simulink model "TriggeredDiagram"  (R2015a)
settings: Solver=FixedStepDiscrete  SolverMode=SingleTasking  StartTime=0.0  StopTime=10.0  FixedStep=1  RelTol=1e-3
settings Model: CovMetricSettings=dwe  CovHtmlReporting=off  covSaveCumulativeToWorkspaceVar=off  CovSaveSingleToWorkspaceVar=off  CovExternalEMLEnable=on  Creator=hbourbou  LastModifiedBy=hbourbou
settings DataIOCC: LimitDataPoints=off  SaveFormat=Dataset
settings DebuggingCC: SFUnexpectedBacktrackingDiag=error  SFNoUnconditionalDefaultTransitionDiag=error
settings HardwareCC: ProdBitPerPointer=64  ProdLargestAtomicFloat=Float  ProdIntDivRoundTo=Zero  ProdEndianess=LittleEndian  ProdHWDeviceType=Specified
settings ModelReferenceCC: PropagateSignalLabelsOutOfModel=on
settings GRTTargetCC: TargetLangStandard=C99 (ISO)  GeneratePreprocessorConditionals=Use local settings

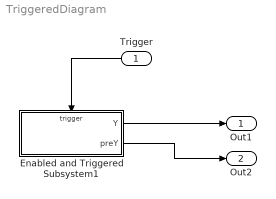
== system TriggeredDiagram ==
  Trigger : Inport  OutDataTypeStr=boolean
  Enabled and Triggered Subsystem1 : Subsystem  TreatAsAtomicUnit=on
  Out1 : Outport
  Out2 : Outport  Port=2
  wires:
  Enabled and Triggered Subsystem1/1(Y) -> Out1/1
  Enabled and Triggered Subsystem1/2(preY) -> Out2/1
  Trigger/1 -> Enabled and Triggered Subsystem1/Trigger

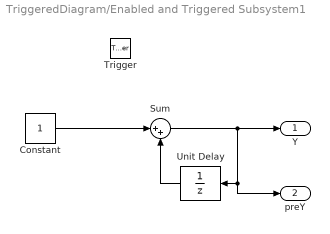
== system TriggeredDiagram/Enabled and Triggered Subsystem1 ==
  Trigger : TriggerPort
  Constant : Constant
  Sum : Sum  Inputs=|++
  Unit Delay : UnitDelay  SampleTime=-1
  Y : Outport  OutputWhenDisabled=reset  InitialOutput=10
  preY : Outport  Port=2  OutputWhenDisabled=reset  InitialOutput=10
  wires:
  Constant/1 -> Sum/1
  Sum/1 -> preY/1, Unit Delay/1, Y/1
  Unit Delay/1 -> Sum/2
